simulink model "LCK_0112"  (R2018b)
settings: Solver=FixedStepDiscrete  StartTime=0.0  StopTime=inf  FixedStep=0.01  RelTol=1e-3
PostLoadFcn:
  | if any(exist('dsrtsu_mdlpostloadfcn', 'file') ~= 0), dsrtsu_mdlpostloadfcn('Execute', bdroot); end
values from neighbouring files (symbols this model uses):
  C_DEG2RAD = 0.0175    [LCK_Macro.sldd]
  C_KPH2MPS = 0.2778    [LCK_Macro.sldd]
  C_NEARZERO = 0.0001    [LCK_Macro.sldd]
  C_ONE = 1.0    [LCK_Macro.sldd]
  C_RAD2DEG = 57.2958    [LCK_Macro.sldd]
  C_ZERO = 0.0    [LCK_Macro.sldd]
  k_accel_pedal_pos_per_speed_x : value not decoded    [LCK_LogicPara.sldd]
  k_accel_pedal_pos_per_speed_z : value not decoded    [LCK_LogicPara.sldd]
  k_brake_suprress_hold = 1000.0    [LCK_LogicPara.sldd]
  k_driver_appl_torque_filt = 50.0    [LCK_LogicPara.sldd]
  k_driver_suppression_hold_time = 3000.0    [LCK_LogicPara.sldd]
  k_hands_on_wheel_hold_msec = 500.0    [LCK_LogicPara.sldd]
  k_hands_on_wheel_torque_hi = 0.2    [LCK_LogicPara.sldd]
  k_hands_on_wheel_torque_lo = 0.15    [LCK_LogicPara.sldd]
  k_handsoff_delay_cycles = 50.0    [LCK_LogicPara.sldd]
  k_handsoff_torq_Lo_CR = 0.3    [LCK_LogicPara.sldd]
  k_handson_delay_cycles = 5.0    [LCK_LogicPara.sldd]
  k_HighAccel_suppress_hold = 3000.0    [LCK_LogicPara.sldd]
  k_HLR_suprress_hold = 3000.0    [LCK_LogicPara.sldd]
  k_hs_StrAng_CR_threshold_z : value not decoded    [LCK_LogicPara.sldd]
  k_LC_Exit_Switch = 0.0    [LCK_LogicPara.sldd]
  k_LCG_Configured = 1.0    [LCK_LogicPara.sldd]
  k_LCK_A0_Rdy2Act_UseConst = 0.0    [LCK_LogicPara.sldd]
  k_LCK_A0Fac_ActSta : value not decoded    [LCK_CtrlPara.sldd]
  k_LCK_A0Fac_DrvStm : value not decoded    [LCK_CtrlPara.sldd]
  k_LCK_A0Shift_LftCurv : value not decoded    [LCK_CtrlPara.sldd]
  k_LCK_A0Shift_RgtCurv : value not decoded    [LCK_CtrlPara.sldd]
  k_LCK_A0Shift_StraLan = 0.0    [LCK_CtrlPara.sldd]
  k_LCK_A0ShiftFac_Dy_LftCurv : value not decoded    [LCK_CtrlPara.sldd]
  k_LCK_A0ShiftFac_Dy_RgtCurv : value not decoded    [LCK_CtrlPara.sldd]
  k_LCK_A0ShiftFac_Vspd : value not decoded    [LCK_CtrlPara.sldd]
  k_LCK_accel_inhibit_thold = 35.0    [LCK_LogicPara.sldd]
  k_LCK_Active2Ready_Mask = 255.0    [LCK_LogicPara.sldd]
  k_LCK_CvatRateBks : value not decoded    [LCK_CtrlPara.sldd]
  k_LCK_CvatrBks : value not decoded    [LCK_CtrlPara.sldd]
  k_LCK_DFac_Dy : value not decoded    [LCK_CtrlPara.sldd]
  k_LCK_DFac_Dy_Curv : value not decoded    [LCK_CtrlPara.sldd]
  k_LCK_DFac_HaCurCen : value not decoded    [LCK_CtrlPara.sldd]
  k_LCK_DFac_HaCurSid : value not decoded    [LCK_CtrlPara.sldd]
  k_LCK_DFac_HadCurCen : value not decoded    [LCK_CtrlPara.sldd]
  k_LCK_DFac_HadCurSid : value not decoded    [LCK_CtrlPara.sldd]
  k_LCK_DFac_HadStrCen : value not decoded    [LCK_CtrlPara.sldd]
  k_LCK_DFac_HadStrSid : value not decoded    [LCK_CtrlPara.sldd]
  k_LCK_DFac_HaStrCen : value not decoded    [LCK_CtrlPara.sldd]
  k_LCK_DFac_HaStrSid : value not decoded    [LCK_CtrlPara.sldd]
  k_LCK_DFac_Rad : value not decoded    [LCK_CtrlPara.sldd]
  k_LCK_DFac_SA_CurCen : value not decoded    [LCK_CtrlPara.sldd]
  k_LCK_DFac_SA_CurSid : value not decoded    [LCK_CtrlPara.sldd]
  k_LCK_DFac_SA_StrCen : value not decoded    [LCK_CtrlPara.sldd]
  k_LCK_DFac_SA_StrSid : value not decoded    [LCK_CtrlPara.sldd]
  k_LCK_DFac_SS_CurCen : value not decoded    [LCK_CtrlPara.sldd]
  k_LCK_DFac_SS_CurSid : value not decoded    [LCK_CtrlPara.sldd]
  k_LCK_DFac_SS_StrCen : value not decoded    [LCK_CtrlPara.sldd]
  k_LCK_DFac_SS_StrSid : value not decoded    [LCK_CtrlPara.sldd]
  k_LCK_DFac_Vspd : value not decoded    [LCK_CtrlPara.sldd]
  k_LCK_DlyTm_DrvStim = 0.2    [LCK_CtrlPara.sldd]
  k_LCK_DTermMax = 2.0    [LCK_CtrlPara.sldd]
  k_LCK_DyBks_Curv : value not decoded    [LCK_CtrlPara.sldd]
  k_LCK_Enable_POOnly = 1.0    [LCK_LogicPara.sldd]
  k_LCK_Entry_DistBuffer = 0.1    [LCK_LogicPara.sldd]
  k_LCK_Fac_Vspd2RngThr_FalRec = 0.23    [LCK_CtrlPara.sldd]
  k_LCK_Ffw_CvatSwh = 0.0    [LCK_CtrlPara.sldd]
  k_LCK_Ffw_DyBks : value not decoded    [LCK_CtrlPara.sldd]
  k_LCK_Ffw_TimCon_CmdFlt = 0.0    [LCK_CtrlPara.sldd]
  k_LCK_FfwDeltaFac_Rad_Lft : value not decoded    [LCK_CtrlPara.sldd]
  k_LCK_FfwDeltaFac_Rad_Rgt : value not decoded    [LCK_CtrlPara.sldd]
  k_LCK_FfwDeltaFac_Vspd : value not decoded    [LCK_CtrlPara.sldd]
  k_LCK_FfwFac_CvatRate_Lft : value not decoded    [LCK_CtrlPara.sldd]
  k_LCK_FfwFac_CvatRate_Rgt : value not decoded    [LCK_CtrlPara.sldd]
  k_LCK_FfwFac_Dy : value not decoded    [LCK_CtrlPara.sldd]
  k_LCK_FfwFac_Rad_Lft : value not decoded    [LCK_CtrlPara.sldd]
  k_LCK_FfwFac_Rad_Rgt : value not decoded    [LCK_CtrlPara.sldd]
  k_LCK_FfwFac_Vspd : value not decoded    [LCK_CtrlPara.sldd]
  k_LCK_FfwTorq_Cvat : value not decoded    [LCK_CtrlPara.sldd]
  k_LCK_HAFac_ActSta : value not decoded    [LCK_CtrlPara.sldd]
  k_LCK_HAFac_DrvStm : value not decoded    [LCK_CtrlPara.sldd]
  k_LCK_HaloTime = 2000.0    [LCK_LogicPara.sldd]
  k_LCK_HaloTime_Switch = 0.0    [LCK_LogicPara.sldd]
  k_LCK_HARFac_ActSta : value not decoded    [LCK_CtrlPara.sldd]
  k_LCK_HARFac_DrvStm : value not decoded    [LCK_CtrlPara.sldd]
  k_LCK_Hed_DyBks : value not decoded    [LCK_CtrlPara.sldd]
  k_LCK_HedAngDiffX : value not decoded    [LCK_CtrlPara.sldd]
  k_LCK_HedAngRateDiffX : value not decoded    [LCK_CtrlPara.sldd]
  k_LCK_HndsOnWhel_DlyTm_Idl2Rdy = 0.0    [LCK_LogicPara.sldd]
  k_LCK_host_veh_width = 1.86    [LCK_LogicPara.sldd]
  k_LCK_Idle2Ready_Mask = 239.0    [LCK_LogicPara.sldd]
  k_LCK_Junc_SusTime = 1.0    [LCK_LogicPara.sldd]
  k_LCK_KpKdDecSlopeLmt = 10.0    [LCK_CtrlPara.sldd]
  k_LCK_KpKdIncSlopeLmt = 5.0    [LCK_CtrlPara.sldd]
  k_LCK_Lat_Ctrl_DFac_Lft = 1.0    [LCK_CtrlPara.sldd]
  k_LCK_Lat_Ctrl_DFac_Rgt = 1.05    [LCK_CtrlPara.sldd]
  k_LCK_Lat_Ctrl_Kd = 0.8    [LCK_CtrlPara.sldd]
  k_LCK_Lat_Ctrl_Ki = 0.5    [LCK_CtrlPara.sldd]
  k_LCK_Lat_Ctrl_Kp = 0.7    [LCK_CtrlPara.sldd]
  k_LCK_Lat_Ctrl_Kp_NearGain = 0.7    [LCK_CtrlPara.sldd]
  k_LCK_Lat_Ctrl_PFac_Lft = 1.0    [LCK_CtrlPara.sldd]
  k_LCK_Lat_Ctrl_PFac_Rgt = 1.05    [LCK_CtrlPara.sldd]
  k_LCK_Lat_Ctrl_TimCon_CmdFlt = 5.0    [LCK_CtrlPara.sldd]
  k_LCK_Lat_DFac_Rad : value not decoded    [LCK_CtrlPara.sldd]
  k_LCK_Lat_DFac_SS_Cur : value not decoded    [LCK_CtrlPara.sldd]
  k_LCK_Lat_DFac_SS_Str : value not decoded    [LCK_CtrlPara.sldd]
  k_LCK_Lat_DFac_Vspd : value not decoded    [LCK_CtrlPara.sldd]
  k_LCK_Lat_DyBks : value not decoded    [LCK_CtrlPara.sldd]
  k_LCK_Lat_IFac_Rad : value not decoded    [LCK_CtrlPara.sldd]
  k_LCK_Lat_IFac_Vspd : value not decoded    [LCK_CtrlPara.sldd]
  k_LCK_Lat_ILmtFac_Dy_CurvLan : value not decoded    [LCK_CtrlPara.sldd]
  k_LCK_Lat_ILmtFac_Dy_StraLan : value not decoded    [LCK_CtrlPara.sldd]
  k_LCK_Lat_ILmtFac_Rad : value not decoded    [LCK_CtrlPara.sldd]
  k_LCK_Lat_ILmtFac_Rad_NearGain = 1.0    [LCK_CtrlPara.sldd]
  k_LCK_Lat_ILmtFac_Vspd_CurvLan : value not decoded    [LCK_CtrlPara.sldd]
  k_LCK_Lat_ILmtFac_Vspd_StraLan : value not decoded    [LCK_CtrlPara.sldd]
  k_LCK_Lat_ITermLmt_Dy = 1.0    [LCK_CtrlPara.sldd]
  k_LCK_Lat_KpKdDecSlopeLmt = 10.0    [LCK_CtrlPara.sldd]
  k_LCK_Lat_KpKdIncSlopeLmt = 10.0    [LCK_CtrlPara.sldd]
  k_LCK_Lat_PFac_Dy_InnLftCur : value not decoded    [LCK_CtrlPara.sldd]
  k_LCK_Lat_PFac_Dy_InnRgtCur : value not decoded    [LCK_CtrlPara.sldd]
  k_LCK_Lat_PFac_Dy_OutLftCur : value not decoded    [LCK_CtrlPara.sldd]
  k_LCK_Lat_PFac_Dy_OutRgtCur : value not decoded    [LCK_CtrlPara.sldd]
  k_LCK_Lat_PFac_Dy_Str : value not decoded    [LCK_CtrlPara.sldd]
  k_LCK_Lat_PFac_Rad : value not decoded    [LCK_CtrlPara.sldd]
  ... (+153 more)
undefined symbols (not defined in the file or in its folder): k_LCK_CurvBks, K_LCK_SPA0A1A2_LMRngCmp_y
libraries: LateralControl_fcns_lib x58, simulink x24
(part 31 of 45)

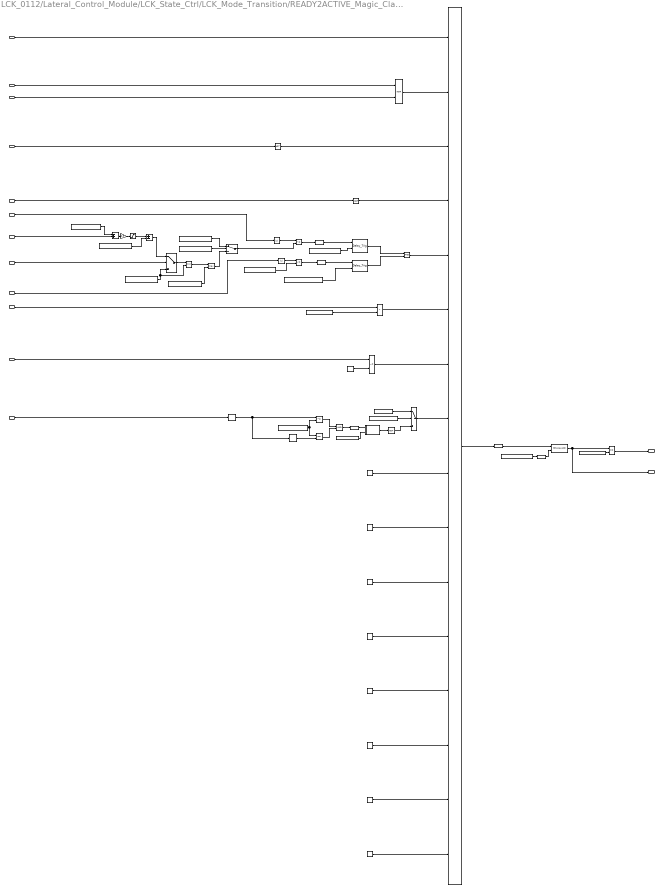
== system LCK_0112/Lateral_Control_Module/LCK_State_Ctrl/LCK_Mode_Transition/READY2ACTIVE_Magic_Claculation ==
  note: Safe distance to lane maker which should be ensured during LCK engage
  note: LKATrqOvrlTrqDStat
      | 0: inactive
      | 1: active
      | 2:Temporary inhibit
      | 3:Permanantly failed
  note: This saturation is only used to filter out negative values
  note: Only when BLM is available and valid is high, can we use the upper branch
  note: Host Vehicle is in the Lane Center
  TJA_LatCtrl_Rq : Inport
  f_driv_override_left : Inport  Port=2
  f_driv_override_right : Inport  Port=3
  f_left_driver_suppression : Inport  Port=4
  f_right_driver_suppression : Inport  Port=5
  SPP_A0 : Inport  Port=6
  curr_lane_width : Inport  Port=7
  SP_valid_high_spd : Inport  Port=8
  SPP_A1 : Inport  Port=9
  ELK_Mode : Inport  Port=10
  LKATrqOvrlTrqDStat : Inport  Port=11
  LCK_Mode : Inport  Port=12
  Abs2 : Abs  Tag={'output',{'type','Float32'},'date',737243.50375769672}  Description=_GWMAB30P3.LCK.000_16_
  Abs5 : Abs  Tag={'output',{'type','Float32'},'date',737243.50381569448}  Description=_GWMAB30P3.LCK.000_17_
  Add2 : Sum  Tag={'output',{'type','Float32'},'date',737531.67944170139}  Description=_GACA26P4.LCK.000_7_  Inputs=-+
  Add3 : Sum  Tag={'output',{'type','Float32'},'date',737531.80311758106}  Description=_GACA26P4.LCK.000_8_  Inputs=+-
  Constant30 : Constant  Tag={'output',{'type','Int32'},'date',737237.63746081013}  Description=_GWMAB30P3.LCK.000_27_  Value=0
  Constant32 : Constant  Tag={'output',{'type','Int32'},'date',737237.63746096066}  Description=_GWMAB30P3.LCK.000_28_  Value=0
  Constant33 : Constant  Tag={'output',{'type','Int32'},'date',737237.63746108802}  Description=_GWMAB30P3.LCK.000_29_  Value=0
  Constant34 : Constant  Tag={'output',{'type','Int32'},'date',737237.6374612269}  Description=_GWMAB30P3.LCK.000_30_  Value=0
  Constant35 : Constant  Tag={'output',{'type','Int32'},'date',737237.63746138883}  Description=_GWMAB30P3.LCK.000_31_  Value=0
  Constant36 : Constant  Tag={'output',{'type','Int32'},'date',737237.63746153936}  Description=_GWMAB30P3.LCK.000_32_  Value=0
  Constant37 : Constant  Tag={'output',{'type','Int32'},'date',737237.63746167824}  Description=_GWMAB30P3.LCK.000_33_  Value=0
  Constant38 : Constant  Tag={'output',{'type','Int32'},'date',737237.63746182865}  Description=_GWMAB30P3.LCK.000_34_  Value=0
  Constant40 : Constant  Tag={'output',{'type','Int32'},'date',737292.69765947922}  Description=_GWMAB30P4.LCK.000_119_  Value=2
  Data Type Conversion14 : DataTypeConversion  Description=_GWMAB30P4.LCK.000_125_  OutDataTypeStr=uint16
  Data Type Conversion32 : DataTypeConversion  Description=_GWMAB30P4.LCK.000_144_
  Data Type Conversion5 : DataTypeConversion  Description=_GWMAB30P4.LCK.000_147_
  Data Type Conversion84 : DataTypeConversion  Description=_GWMH9P4.LCK.000_68_
  Data Type Conversion94 : DataTypeConversion  OutDataTypeStr=uint16
  Delay : Delay  DelayLength=1  InitialCondition=0
  Delay1 : Delay  DelayLength=1  InitialCondition=0
  Delay_Trig : LateralControl_fcns_lib/Delay_Trig  SystemSampleTime=-1
  Delay_Trig1 : LateralControl_fcns_lib/Delay_Trig  SystemSampleTime=-1
  ELK_MODE_STAGE1_LEFT : Constant  Tag={'output',{'name','$P','class','EXTERN_MACRO','type','ESR_Typedefs/ELK_Mode_T'},'date',737293.52375928243}  Description=_GWMAB30P4.LCK.000_174_  Value=10
  Gain18 : Gain  Tag={'output',{'type','Float32'},'gain',{'type','Int32'},'date',737531.67949780088}  Description=_GACA26P4.LCK.000_15_  Gain=0.5
  Idle2ReadyBitwise 1 : simulink/Logic and Bit Operations/Bitwise Operator  logicop=AND  UseBitMask=off  NumInputPorts=2  BitMask=k_LCK_Ready2Idle_Mask  BitMaskRealWorld=Stored Integer
  LCK_HaloTime_Expired : Constant  Tag={'output',{'type','Int32'},'date',737462.50907098374}  Description=_GWMH9P4.LCK.000_87_
  LCK_MODE_ACTIVE2 : Constant  Tag={'output',{'name','$P','class','EXTERN_MACRO','type','UInt8'},'date',737462.71846480318}  Description=_GWMH9P4.LCK.000_88_  Value=LCK_MODE_ACTIVE
  Logical Operator26 : Logic  Tag={'date',737237.6374667593}  Description=_GWMAB30P3.LCK.000_63_  AllPortsSameDT=off  OutDataTypeStr=boolean
  Logical Operator58 : Logic  Tag={'date',737237.6374691088}  Description=_GWMAB30P3.LCK.000_76_  Operator=NOR  AllPortsSameDT=off  OutDataTypeStr=boolean
  Logical Operator64 : Logic  Tag={'date',737237.63746982638}  Description=_GWMAB30P3.LCK.000_81_  Operator=NOT  Inputs=1  AllPortsSameDT=off  OutDataTypeStr=boolean
  Logical Operator65 : Logic  Tag={'date',737237.63746995374}  Description=_GWMAB30P3.LCK.000_82_  Operator=NOT  Inputs=1  AllPortsSameDT=off  OutDataTypeStr=boolean
  Logical Operator86 : Logic  Tag={'date',737462.50908469909}  Description=_GWMH9P4.LCK.000_126_  AllPortsSameDT=off  OutDataTypeStr=boolean
  Logical Operator93 : Logic  Tag={'date',737462.5090854282}  Description=_GWMH9P4.LCK.000_128_  Operator=NOT  AllPortsSameDT=off  OutDataTypeStr=boolean
  MinMax1 : MinMax  Tag={'output',{'type','Float32'},'date',737531.79481781251}  Description=_GACA26P4.LCK.000_33_  Inputs=2
  MinMax2 : MinMax  Tag={'output',{'type','Float32'},'date',737531.79497368052}  Description=_GACA26P4.LCK.000_34_  Function=max  Inputs=2
  READY2ACTIVE_Magic : LateralControl_fcns_lib/Bit_To_Integer_16  SystemSampleTime=-1
  Ready2Active_Mask1 : Constant  Description=_GWMH9P4.LCK.000_131_  Value=k_LCK_Ready2Active_Mask  SampleTime=-1
  Relational Operator12 : RelationalOperator  Tag={'date',737292.6976643519}  Description=_GWMAB30P4.LCK.000_180_  Operator=<  OutDataTypeStr=boolean  RndMeth=Nearest
  Relational Operator16 : RelationalOperator  Tag={'date',737237.63747063652}  Description=_GWMAB30P3.LCK.000_85_  Operator=<=  OutDataTypeStr=boolean  RndMeth=Nearest
  Relational Operator17 : RelationalOperator  Tag={'date',737237.63747076388}  Description=_GWMAB30P3.LCK.000_86_  Operator=<=  OutDataTypeStr=boolean  RndMeth=Nearest
  Relational Operator19 : RelationalOperator  Tag={'date',737292.69766489579}  Description=_GWMAB30P4.LCK.000_182_  Operator=~=  OutDataTypeStr=boolean  RndMeth=Nearest
  Relational Operator199 : RelationalOperator  Tag={'date',737462.50909643515}  Description=_GWMH9P4.LCK.000_134_  Operator===  OutDataTypeStr=boolean  RndMeth=Nearest
  Relational Operator99 : RelationalOperator  Tag={'date',737462.50910348375}  Description=_GWMH9P4.LCK.000_140_  Operator=~=  OutDataTypeStr=boolean  RndMeth=Nearest
  Relational_Operator2 : RelationalOperator  Tag={'date',737237.63747429394}  Description=_GWMAB30P3.LCK.000_105_  Operator===  OutDataTypeStr=boolean  RndMeth=Nearest
  Saturation : Saturate  Tag={'output',{'type','Float32'},'lowerlimit',{'type','Int32'},'upperlimit',{'type','Int32'},'date',737531.67964041664}  Description=_GACA26P4.LCK.000_42_  UpperLimit=10  LowerLimit=0
  Switch62 : Switch  Tag={'output',{'type','Bool'},'threshold',{'type','Int32'},'date',737463.80756756943}  Description=_GWMH9P4.LCK.000_150_  Threshold=0.5
  Switch65 : Switch  Tag={'output',{'type','Float32'},'threshold',{'type','Int32'},'date',737531.8031876157}  Description=_GACA26P4.LCK.000_45_  Criteria=u2 > Threshold  Threshold=0.5
  Switch66 : Switch  Tag={'output',{'type','Float32'},'threshold',{'type','Int32'},'date',737531.80919148144}  Description=_GACA26P4.LCK.000_46_  Criteria=u2 > Threshold  Threshold=0.5
  Trigger Hold2 : Subsystem
  k_LCK_Entry_DistBuffer : Constant  Tag={'output',{'name','$P','class','EXTERN_CAL','type','Float32'},'date',737531.80306754634}  Description=_GACA26P4.LCK.000_58_  Value=k_LCK_Entry_DistBuffer
  k_LCK_HaloTime : Constant  Tag={'output',{'name','$P','class','EXTERN_CAL','type','UInt16'},'date',737464.62979534722}  Description=_GWMH9P4.LCK.000_174_  Value=k_LCK_HaloTime
  k_LCK_HaloTime_Switch : Constant  Tag={'output',{'name','$P','class','EXTERN_CAL','type','Bool'},'date',737464.6274484375}  Description=_GWMH9P4.LCK.000_175_  Value=k_LCK_HaloTime_Switch
  k_LCK_LnCetr_DlyTm_Rdy2Act : Constant  Tag={'output',{'name','$P','class','EXTERN_CAL','type','Float32'},'date',737464.62610440969}  Description=_GWMAB30P3.LCK.000_134_  Value=k_LCK_LnCetr_DlyTm_Rdy2Act
  k_LCK_LnCetr_DlyTm_Rdy2Act1 : Constant  Tag={'output',{'name','$P','class','EXTERN_CAL','type','Float32'},'date',737464.62635827542}  Description=_GWMAB30P3.LCK.000_135_  Value=k_LCK_LnCetr_DlyTm_Rdy2Act
  k_LCK_Ready2Active_Mask : Constant  Value=k_LCK_Ready2Active_Mask
  k_LCK_SP_A0_Rdy2Act1 : Constant  Tag={'output',{'name','$P','class','EXTERN_CAL','type','Float32'},'date',737531.7947690509}  Description=_GACA26P4.LCK.000_63_  Value=k_LCK_SP_A0_Rdy2Act_Max
  k_LCK_SP_A0_Rdy2Act2 : Constant  Tag={'output',{'name','$P','class','EXTERN_CAL','type','Float32'},'date',737531.79501248838}  Description=_GACA26P4.LCK.000_64_  Value=k_LCK_SP_A0_Rdy2Act_Min
  k_LCK_SP_A0_Rdy2Act3 : Constant  Tag={'output',{'name','$P','class','EXTERN_CAL','type','Bool'},'date',737531.63814517367}  Description=_GACA26P4.LCK.000_65_  Value=k_LCK_A0_Rdy2Act_UseConst
  k_LCK_SP_A0_Rdy2Act4 : Constant  Tag={'output',{'name','$P','class','EXTERN_CAL','type','Float32'},'date',737531.6382341088}  Description=_GACA26P4.LCK.000_66_  Value=k_LCK_SP_A0_Rdy2Act
  k_LCK_SP_A1_Rdy2Act : Constant  Tag={'output',{'name','$P','class','EXTERN_CAL','type','Float32'},'date',737246.86453234951}  Description=_GWMAB30P3.LCK.000_142_  Value=k_LCK_SP_A1_Rdy2Act
  k_LCK_host_veh_width : Constant  Tag={'output',{'name','$P','class','EXTERN_CAL','type','Float32'},'date',737531.63869547448}  Description=_GACA26P4.LCK.000_72_  Value=k_LCK_host_veh_width
  READY2ACTIVE_Magic_Out : Outport
  READY2ACTIVE : Outport  Port=2
  wires:
  Switch62/1 -> READY2ACTIVE_Magic/8
  Constant32/1 -> READY2ACTIVE_Magic/9
  k_LCK_Ready2Active_Mask/1 -> Data Type Conversion94/1
  Gain18/1 -> Saturation/1
  k_LCK_LnCetr_DlyTm_Rdy2Act1/1 -> Delay_Trig1/2
  k_LCK_host_veh_width/1 -> Add2/1
  k_LCK_SP_A0_Rdy2Act2/1 -> MinMax2/2
  READY2ACTIVE_Magic/1 -> Data Type Conversion14/1
  Data Type Conversion84/1 -> Trigger Hold2/1(Trigger)
  Constant40/1 -> Relational Operator19/2
  Abs5/1 -> Relational Operator17/1
  Data Type Conversion14/1 -> Idle2ReadyBitwise 1/1
  k_LCK_SP_A0_Rdy2Act4/1 -> Switch66/1
  Relational Operator19/1 -> READY2ACTIVE_Magic/7
  Data Type Conversion94/1 -> Idle2ReadyBitwise 1/2
  Relational Operator99/1 -> Logical Operator86/1
  Logical Operator64/1 -> READY2ACTIVE_Magic/3
  Logical Operator26/1 -> READY2ACTIVE_Magic/5
  Logical Operator58/1 -> READY2ACTIVE_Magic/2
  Abs2/1 -> Relational Operator16/1
  Data Type Conversion32/1 -> Delay_Trig/1
  Delay_Trig/1 -> Logical Operator26/1
  Constant38/1 -> READY2ACTIVE_Magic/15
  k_LCK_SP_A1_Rdy2Act/1 -> Relational Operator17/2
  Relational Operator17/1 -> Data Type Conversion5/1
  Add2/1 -> Gain18/1
  Constant33/1 -> READY2ACTIVE_Magic/12
  LCK_MODE_ACTIVE2/1 -> Relational Operator199/1, Relational Operator99/2
  Relational_Operator2/1 -> READY2ACTIVE/1
  Add3/1 -> Switch65/1
  LCK_Mode/1 -> Delay1/1
  Constant34/1 -> READY2ACTIVE_Magic/13
  Ready2Active_Mask1/1 -> Relational_Operator2/2
  f_left_driver_suppression/1 -> Logical Operator64/1
  k_LCK_LnCetr_DlyTm_Rdy2Act/1 -> Delay_Trig/2
  Switch66/1 -> Relational Operator16/2
  k_LCK_SP_A0_Rdy2Act3/1 -> Switch66/2
  Constant35/1 -> READY2ACTIVE_Magic/16
  Delay_Trig1/1 -> Logical Operator26/2
  Logical Operator65/1 -> READY2ACTIVE_Magic/4
  ELK_MODE_STAGE1_LEFT/1 -> Relational Operator12/2
  Data Type Conversion5/1 -> Delay_Trig1/1
  k_LCK_HaloTime_Switch/1 -> Switch62/2
  Delay/1 -> Relational Operator199/2
  Constant36/1 -> READY2ACTIVE_Magic/11
  Switch65/1 -> MinMax1/1
  Constant37/1 -> READY2ACTIVE_Magic/14
  Idle2ReadyBitwise 1/1 -> READY2ACTIVE_Magic_Out/1, Relational_Operator2/1
  Relational Operator199/1 -> Logical Operator86/2
  Relational Operator16/1 -> Data Type Conversion32/1
  MinMax2/1 -> Switch66/3
  Relational Operator12/1 -> READY2ACTIVE_Magic/6
  Logical Operator93/1 -> Switch62/3
  k_LCK_Entry_DistBuffer/1 -> Add3/2
  Saturation/1 -> Add3/1
  LCK_HaloTime_Expired/1 -> Switch62/1
  MinMax1/1 -> MinMax2/1
  Trigger Hold2/1(Out) -> Logical Operator93/1
  SP_valid_high_spd/1 -> Switch65/2
  k_LCK_SP_A0_Rdy2Act1/1 -> Switch65/3, MinMax1/2
  k_LCK_HaloTime/1 -> Trigger Hold2/2(hold_time)
  Constant30/1 -> READY2ACTIVE_Magic/10
  Logical Operator86/1 -> Data Type Conversion84/1
  SPP_A1/1 -> Abs5/1
  f_right_driver_suppression/1 -> Logical Operator65/1
  f_driv_override_left/1 -> Logical Operator58/1
  f_driv_override_right/1 -> Logical Operator58/2
  curr_lane_width/1 -> Add2/2
  LKATrqOvrlTrqDStat/1 -> Relational Operator19/1
  TJA_LatCtrl_Rq/1 -> READY2ACTIVE_Magic/1
  ELK_Mode/1 -> Relational Operator12/1
  SPP_A0/1 -> Abs2/1
  Delay1/1 -> Delay/1, Relational Operator99/1
